simulink model "qimozuoye"  (R2015a)
settings: Solver=ode23tb  StartTime=0.0  StopTime=5  RelTol=1e-3
libraries: powerlib x12, powerlib_extras x3
settings Model: Creator=Administrator  LastModifiedBy=佳君
settings DataIOCC: SignalLoggingSaveFormat=ModelDataLogs
settings OptimizationCC: ExpressionDepthLimit=2147483647
settings DebuggingCC: UnderspecifiedInitializationDetection=Classic  MergeDetectMultiDrivingBlocksExec=none  SolverPrmCheckMsg=warning  FcnCallInpInsideContextMsg=UseLocalSettings  StateNameClashWarn=warning  StrictBusMsg=Warning
settings GRTTargetCC: CombineOutputUpdateFcns=off  GRTInterface=on

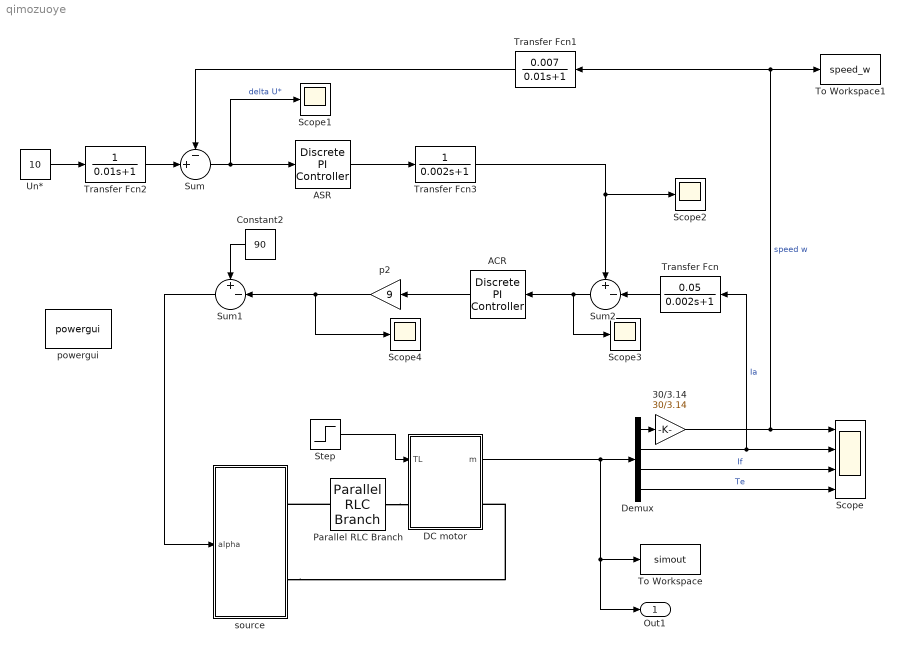
== system qimozuoye ==
  30/3.14 : Gain  Gain=30/3.14
  ACR : powerlib_extras/Discrete  Control Blocks/Discrete PI Controller  Kp=1.013  Ki=33.77  Par_Limits=[10 0]  Init=0  Ts=50e-6
  ASR : powerlib_extras/Discrete  Control Blocks/Discrete PI Controller  Kp=11.7  Ki=134  Par_Limits=[10 0]  Init=0  Ts=50e-6
  Constant2 : Constant  Value=90
  DC motor : Subsystem
  Demux : Demux
  Parallel RLC Branch : powerlib/Elements/Parallel RLC Branch  LConnTagsString=a  RConnTagsString=__new0  BranchType=L  Resistance=1  Inductance=1e-3  SetiL0=off  InitialCurrent=0  Capacitance=1e-6  Setx0=off  InitialVoltage=0  Measurements=Branch voltage and current
  Scope : Scope  NumInputPorts=4
      settings: TimeRange=5  YMin=0~-50~0.870837~-100  YMax=2000~250~0.962503~300
  Scope{1..4} (4 alike) : Scope
      Scope1 settings: YMin=-0.5  YMax=1
      Scope2 settings: YMin=0  YMax=25  SaveName=ScopeData2
      Scope3 settings: YMin=-0.5  YMax=1  SaveName=ScopeData3
      Scope4 settings: YMin=-0.5  YMax=1  SaveName=ScopeData4
  Step : Step  Time=2  Before=80  After=100  SampleTime=0
  Sum : Sum  Inputs=-+|
  Sum1 : Sum  Inputs=+-|
  Sum2 : Sum  Inputs=+-|
  To Workspace : ToWorkspace  VariableName=simout  SaveFormat=Structure  SampleTime=-1
  To Workspace1 : ToWorkspace  VariableName=speed_w  SaveFormat=Structure With Time  SampleTime=-1
  Transfer Fcn : TransferFcn  Numerator=[0.05]  Denominator=[0.002 1]
  Transfer Fcn1 : TransferFcn  Numerator=[0.007]  Denominator=[0.01 1]
  Transfer Fcn2 : TransferFcn  Denominator=[0.01 1]
  Transfer Fcn3 : TransferFcn  Denominator=[0.002 1]
  Un* : Constant  Value=10
  p2 : Gain  Gain=9
  powergui : powerlib/powergui  Priority=1  SimulationMode=Continuous  SolverType=Tustin/Backward Euler (TBE)  SampleTime=50e-6  frequency=60  SPID=off  DisableSnubberDevices=off  DisableRonSwitches=off  DisableVfSwitches=off  SwTol=0  DisplayEquations=off  Interpol=off  methode=off  Ts=0  FunctionMessages=off  echomessages=off  HookPort=off  EnableUseOfTLC=off  x0status=blocks  frequencyindice=0  Pbase=100e6  ErrMax=1e-4  Iterations=50  UnitsV=kV  UnitsW=MW  buscounter=0  RestoreLinks=warning  ResistiveCurrentMeasurement=off  Frange=[0:2:500]  Ylog=off  Xlog=on  ShowGrid=off  save=off  variable=ZData  structure=0  ZoomFFT=on  StartTime=0.0  cycles=1  DisplayStyle=1  fundamental=60  FreqAxis=off  MaxFrequency=1000  frequencyindicesteady=1  RmsSteady=1  display=off
  source : Subsystem
  Out1 : Outport
  wires:
  DC motor/1(m) -> Demux/1, Out1/1, To Workspace/1
  Demux/2 -> Transfer Fcn/1, Scope/2  "Ia"
  Demux/3 -> Scope/3  "If"
  Demux/4 -> Scope/4  "Te"
  Demux/1 -> 30/3.14/1
  Un*/1 -> Transfer Fcn2/1
  30/3.14/1 -> Scope/1, Transfer Fcn1/1, To Workspace1/1  "speed w"
  Transfer Fcn1/1 -> Sum/1
  Sum/1 -> Scope1/1, ASR/1  "delta U*"
  Constant2/1 -> Sum1/1
  Step/1 -> DC motor/1(TL)
  Transfer Fcn/1 -> Sum2/2
  Sum2/1 -> Scope3/1, ACR/1
  Transfer Fcn3/1 -> Scope2/1, Sum2/1
  ACR/1 -> p2/1
  p2/1 -> Sum1/2, Scope4/1
  Transfer Fcn2/1 -> Sum/2
  ASR/1 -> Transfer Fcn3/1
  Sum1/1 -> source/1(alpha)
  connections:
  Parallel RLC Branch/LConn1 -- source/RConn1
  source/RConn2 -- DC motor/RConn1
  Parallel RLC Branch/RConn1 -- DC motor/LConn1

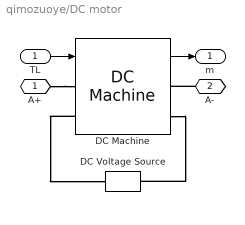
== system qimozuoye/DC motor ==
  TL : Inport
  DC Machine : powerlib/Machines/DC Machine  PresetModel=No  MechanicalLoad=Torque TL  FieldType=Wound  ShowDetailedParameters=on  MeasurementBus=off  RLa=[0.2 0.015]  RLf=[240 120]  Laf=1.376  MachineConstant=Torque constant (N.m/A)  Ke=1.8  Kt=1.8  J=0.573  Bm=0  Tf=0  w0=1  Ifinit=0.91666666666666666666666666666666666666  TsPowergui=0  TsBlock=-1
  DC Voltage Source : powerlib/Electrical Sources/DC Voltage Source  Amplitude=220  Measurements=None
  A+ : PMIOPort  Port=1  Side=Left
  A- : PMIOPort  Port=2  Side=Right
  m : Outport
  wires:
  TL/1 -> DC Machine/1
  DC Machine/1 -> m/1
  connections:
  DC Machine/LConn2 -- DC Voltage Source/RConn1
  DC Machine/RConn2 -- DC Voltage Source/LConn1
  A+/RConn1 -- DC Machine/LConn1
  A-/RConn1 -- DC Machine/RConn1

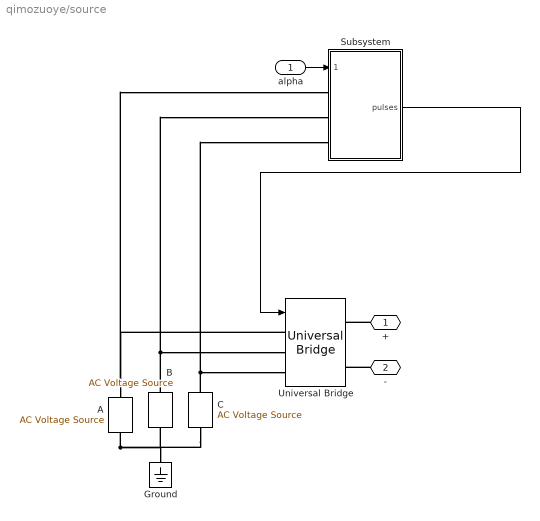
== system qimozuoye/source ==
  alpha : Inport
  A : powerlib/Electrical Sources/AC Voltage Source  Amplitude=220  Phase=0  Frequency=50  SampleTime=0  Measurements=Voltage
  B : powerlib/Electrical Sources/AC Voltage Source  Amplitude=220  Phase=240  Frequency=50  SampleTime=0  Measurements=Voltage
  C : powerlib/Electrical Sources/AC Voltage Source  Amplitude=220  Phase=120  Frequency=50  SampleTime=0  Measurements=Voltage
  Ground : powerlib/Elements/Ground  LConnTagsString=a
  Subsystem : Subsystem
  Universal Bridge : powerlib/Power Electronics/Universal Bridge  Arms=3  SnubberResistance=1e5  SnubberCapacitance=inf  Device=Thyristors  Ron=0.3  Lon=0  ForwardVoltages="[  0  0  ]"  ForwardVoltage=0  GTOparameters=[ 10e-6 , 20e-6 ]  IGBTparameters=[ 1e-6 , 2e-6 ]  Measurements=None  Measurements_2=None  converterType=Rectifier
  + : PMIOPort  Port=1  Side=Right
  - : PMIOPort  Port=2  Side=Right
  wires:
  Subsystem/1(pulses) -> Universal Bridge/1
  alpha/1 -> Subsystem/1(alpha_deg)
  connections:
  A/LConn1 -- C/LConn1 -- B/LConn1 -- Ground/LConn1
  A/RConn1 -- Subsystem/LConn1 -- Universal Bridge/LConn1
  B/RConn1 -- Subsystem/LConn2 -- Universal Bridge/LConn2
  C/RConn1 -- Subsystem/LConn3 -- Universal Bridge/LConn3
  +/RConn1 -- Universal Bridge/RConn1
  -/RConn1 -- Universal Bridge/RConn2

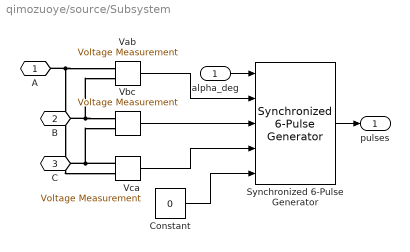
== system qimozuoye/source/Subsystem ==
  alpha_deg : Inport
  Constant : Constant  Value=0
  Synchronized 6-Pulse Generator : powerlib_extras/Control  Blocks/Synchronized 6-Pulse Generator  freq=50  pwidth=10  Double_Pulse=off
  Vab : powerlib/Measurements/Voltage Measurement  PhasorSimulation=off  OutputType=Complex  PSBequivalent=0
  Vbc : powerlib/Measurements/Voltage Measurement  PhasorSimulation=off  OutputType=Complex  PSBequivalent=0
  Vca : powerlib/Measurements/Voltage Measurement  PhasorSimulation=off  OutputType=Complex  PSBequivalent=0
  A : PMIOPort  Port=1  Side=Left
  B : PMIOPort  Port=2  Side=Left
  C : PMIOPort  Port=3  Side=Left
  pulses : Outport
  wires:
  Vab/1 -> Synchronized 6-Pulse Generator/2
  Vbc/1 -> Synchronized 6-Pulse Generator/3
  Vca/1 -> Synchronized 6-Pulse Generator/4
  Constant/1 -> Synchronized 6-Pulse Generator/5
  alpha_deg/1 -> Synchronized 6-Pulse Generator/1
  Synchronized 6-Pulse Generator/1 -> pulses/1
  connections:
  A/RConn1 -- Vca/LConn2 -- Vab/LConn1
  B/RConn1 -- Vbc/LConn1 -- Vab/LConn2
  C/RConn1 -- Vca/LConn1 -- Vbc/LConn2
